simulink model "SigProcess"  (R2022b)
settings: Solver=FixedStepDiscrete  StartTime=0.0  StopTime=10.0  FixedStep=0.001  RelTol=1e-3
undefined symbols (not defined in the file): cClCddAdc_D_u16ADNum, cClCddAdc_D_u8FilterType, cClCddAdc_D_u8RawValueNum, cTmAfCtrl_Te_s32ShttrPosnColdOnHp
libraries: simulink x132
(part 5 of 7)

== system SigProcess/SigProcessSub/Stp6_createPortGotoUpdate/CLHB02001_AdFilter/AVG6 ==
  sigin : Inport
  Compare To Constant : simulink/Logic and Bit Operations/Compare To Constant  relop===  const=0  OutDataTypeStr=boolean
  Constant : Constant  Value=cClCddAdc_D_u8FilterType  OutDataTypeStr=uint8
  Constant1 : Constant  Value=cClCddAdc_D_u8RawValueNum  OutDataTypeStr=uint8
  Counter Limited : simulink/Sources/Counter Limited  uplimit=cClCddAdc_D_u8RawValueNum-1  tsamp=-1
  Data Store Memory : DataStoreMemory  DataStoreName=TempFlapFroLiFbRaw  ReadBeforeWriteMsg=warning  WriteAfterWriteMsg=warning  WriteAfterReadMsg=warning  ShowAdditionalParam=off  OutDataTypeStr=single  Dimensions=[1 20]
      settings: CopyFcn=set_param(gcbh,'ShowName','off');
  Data Store Read : DataStoreRead  DataStoreName=TempFlapFroLiFbRaw  IndexOptions=Index vector (dialog)  Indices=1  OutputSizes=1
  Data Store Write : DataStoreWrite  DataStoreName=TempFlapFroLiFbRaw  DataStoreElements=TempFlapFroLiFbRaw  EnableIndexing=on  IndexMode=Zero-based  IndexOptions=Index vector (port)  Indices=1  OutputSizes=1
  Data Type Conversion : DataTypeConversion  OutDataTypeStr=single  SaturateOnIntegerOverflow=off  RndMeth=Floor
  Gain1 : Gain  Gain=1/cClCddAdc_D_u8RawValueNum
  MATLAB Function : MATLAB Function  TreatAsAtomicUnit=on
  Multiport Switch : MultiPortSwitch  DataPortOrder=Zero-based contiguous  Inputs=5  DataPortForDefault=Additional data port  zeroidx=on  OutDataTypeStr=single  SaturateOnIntegerOverflow=off  InputSameDT=off
  Scope : Scope
  Sum of Elements1 : Sum  Inputs=+
  Switch : Switch  Criteria=u2 ~= 0  SaturateOnIntegerOverflow=off  InputSameDT=off
  Unit Delay : UnitDelay  SampleTime=-1  HasFrameUpgradeWarning=on
  sigAvg : Outport  OutDataTypeStr=single
  wires:
  Data Store Read/1 -> MATLAB Function/1(u), Sum of Elements1/1
  Sum of Elements1/1 -> Gain1/1
  Compare To Constant/1 -> Switch/2
  Switch/1 -> [sigAvgSimple], Unit Delay/1
  Gain1/1 -> Switch/1, [sigAvgQuick]
  Counter Limited/1 -> Compare To Constant/1, Data Store Write/2
  Data Type Conversion/1 -> [siginSingle], Data Store Write/1, Scope/1
  MATLAB Function/2(withoutEdge) -> [sigAvgSortWithoutEdge]
  Unit Delay/1 -> Switch/3
  MATLAB Function/1(mid) -> [sigAvgSortedMid]
  sigin/1 -> [sigin]
  [sigin] -> Data Type Conversion/1
  [sigin] -> Multiport Switch/7
  Constant/1 -> Multiport Switch/1
  [sigAvgSortedMid] -> Multiport Switch/3
  [sigAvgSortWithoutEdge] -> Multiport Switch/4
  [sigAvgSimple] -> Multiport Switch/5
  [sigAvgQuick] -> Multiport Switch/6
  [siginSingle] -> Multiport Switch/2
  Multiport Switch/1 -> [sigAvg]
  [sigAvg] -> sigAvg/1
  Constant1/1 -> MATLAB Function/2(num)

== system SigProcess/SigProcessSub/Stp6_createPortGotoUpdate/CLHB02001_AdFilter/AVG7 ==
  sigin : Inport
  Compare To Constant : simulink/Logic and Bit Operations/Compare To Constant  relop===  const=0  OutDataTypeStr=boolean
  Constant : Constant  Value=cClCddAdc_D_u8FilterType  OutDataTypeStr=uint8
  Constant1 : Constant  Value=cClCddAdc_D_u8RawValueNum  OutDataTypeStr=uint8
  Counter Limited : simulink/Sources/Counter Limited  uplimit=cClCddAdc_D_u8RawValueNum-1  tsamp=-1
  Data Store Memory : DataStoreMemory  DataStoreName=TempFlapFroRIFbRaw  ReadBeforeWriteMsg=warning  WriteAfterWriteMsg=warning  WriteAfterReadMsg=warning  ShowAdditionalParam=off  OutDataTypeStr=single  Dimensions=[1 20]
      settings: CopyFcn=set_param(gcbh,'ShowName','off');
  Data Store Read : DataStoreRead  DataStoreName=TempFlapFroRIFbRaw  IndexOptions=Index vector (dialog)  Indices=1  OutputSizes=1
  Data Store Write : DataStoreWrite  DataStoreName=TempFlapFroRIFbRaw  DataStoreElements=TempFlapFroRIFbRaw  EnableIndexing=on  IndexMode=Zero-based  IndexOptions=Index vector (port)  Indices=1  OutputSizes=1
  Data Type Conversion : DataTypeConversion  OutDataTypeStr=single  SaturateOnIntegerOverflow=off  RndMeth=Floor
  Gain1 : Gain  Gain=1/cClCddAdc_D_u8RawValueNum
  MATLAB Function : MATLAB Function  TreatAsAtomicUnit=on
  Multiport Switch : MultiPortSwitch  DataPortOrder=Zero-based contiguous  Inputs=5  DataPortForDefault=Additional data port  zeroidx=on  OutDataTypeStr=single  SaturateOnIntegerOverflow=off  InputSameDT=off
  Scope : Scope
  Sum of Elements1 : Sum  Inputs=+
  Switch : Switch  Criteria=u2 ~= 0  SaturateOnIntegerOverflow=off  InputSameDT=off
  Unit Delay : UnitDelay  SampleTime=-1  HasFrameUpgradeWarning=on
  sigAvg : Outport  OutDataTypeStr=single
  wires:
  Constant1/1 -> MATLAB Function/2(num)
  [sigAvg] -> sigAvg/1
  Multiport Switch/1 -> [sigAvg]
  [siginSingle] -> Multiport Switch/2
  [sigAvgQuick] -> Multiport Switch/6
  [sigAvgSimple] -> Multiport Switch/5
  [sigAvgSortWithoutEdge] -> Multiport Switch/4
  [sigAvgSortedMid] -> Multiport Switch/3
  Constant/1 -> Multiport Switch/1
  [sigin] -> Multiport Switch/7
  [sigin] -> Data Type Conversion/1
  sigin/1 -> [sigin]
  MATLAB Function/1(mid) -> [sigAvgSortedMid]
  Unit Delay/1 -> Switch/3
  MATLAB Function/2(withoutEdge) -> [sigAvgSortWithoutEdge]
  Data Type Conversion/1 -> Scope/1, Data Store Write/1, [siginSingle]
  Counter Limited/1 -> Data Store Write/2, Compare To Constant/1
  Gain1/1 -> [sigAvgQuick], Switch/1
  Switch/1 -> Unit Delay/1, [sigAvgSimple]
  Compare To Constant/1 -> Switch/2
  Sum of Elements1/1 -> Gain1/1
  Data Store Read/1 -> Sum of Elements1/1, MATLAB Function/1(u)

== system SigProcess/SigProcessSub/Stp6_createPortGotoUpdate/CLHB02001_AdFilter/AVG8 ==
  sigin : Inport
  Compare To Constant : simulink/Logic and Bit Operations/Compare To Constant  relop===  const=0  OutDataTypeStr=boolean
  Constant : Constant  Value=cClCddAdc_D_u8FilterType  OutDataTypeStr=uint8
  Constant1 : Constant  Value=cClCddAdc_D_u8RawValueNum  OutDataTypeStr=uint8
  Counter Limited : simulink/Sources/Counter Limited  uplimit=cClCddAdc_D_u8RawValueNum-1  tsamp=-1
  Data Store Memory : DataStoreMemory  DataStoreName=ModFlapFroRIFbRaw  ReadBeforeWriteMsg=warning  WriteAfterWriteMsg=warning  WriteAfterReadMsg=warning  ShowAdditionalParam=off  OutDataTypeStr=single  Dimensions=[1 20]
      settings: CopyFcn=set_param(gcbh,'ShowName','off');
  Data Store Read : DataStoreRead  DataStoreName=ModFlapFroRIFbRaw  IndexOptions=Index vector (dialog)  Indices=1  OutputSizes=1
  Data Store Write : DataStoreWrite  DataStoreName=ModFlapFroRIFbRaw  DataStoreElements=ModFlapFroRIFbRaw  EnableIndexing=on  IndexMode=Zero-based  IndexOptions=Index vector (port)  Indices=1  OutputSizes=1
  Data Type Conversion : DataTypeConversion  OutDataTypeStr=single  SaturateOnIntegerOverflow=off  RndMeth=Floor
  Gain1 : Gain  Gain=1/cClCddAdc_D_u8RawValueNum
  MATLAB Function : MATLAB Function  TreatAsAtomicUnit=on
  Multiport Switch : MultiPortSwitch  DataPortOrder=Zero-based contiguous  Inputs=5  DataPortForDefault=Additional data port  zeroidx=on  OutDataTypeStr=single  SaturateOnIntegerOverflow=off  InputSameDT=off
  Scope : Scope
  Sum of Elements1 : Sum  Inputs=+
  Switch : Switch  Criteria=u2 ~= 0  SaturateOnIntegerOverflow=off  InputSameDT=off
  Unit Delay : UnitDelay  SampleTime=-1  HasFrameUpgradeWarning=on
  sigAvg : Outport  OutDataTypeStr=single
  wires:
  Data Store Read/1 -> MATLAB Function/1(u), Sum of Elements1/1
  Sum of Elements1/1 -> Gain1/1
  Compare To Constant/1 -> Switch/2
  Switch/1 -> [sigAvgSimple], Unit Delay/1
  Gain1/1 -> Switch/1, [sigAvgQuick]
  Counter Limited/1 -> Compare To Constant/1, Data Store Write/2
  Data Type Conversion/1 -> [siginSingle], Data Store Write/1, Scope/1
  MATLAB Function/2(withoutEdge) -> [sigAvgSortWithoutEdge]
  Unit Delay/1 -> Switch/3
  MATLAB Function/1(mid) -> [sigAvgSortedMid]
  sigin/1 -> [sigin]
  [sigin] -> Data Type Conversion/1
  [sigin] -> Multiport Switch/7
  Constant/1 -> Multiport Switch/1
  [sigAvgSortedMid] -> Multiport Switch/3
  [sigAvgSortWithoutEdge] -> Multiport Switch/4
  [sigAvgSimple] -> Multiport Switch/5
  [sigAvgQuick] -> Multiport Switch/6
  [siginSingle] -> Multiport Switch/2
  Multiport Switch/1 -> [sigAvg]
  [sigAvg] -> sigAvg/1
  Constant1/1 -> MATLAB Function/2(num)

== system SigProcess/SigProcessSub/Stp6_createPortGotoUpdate/CLHB02001_AdFilter/AVG9 ==
  sigin : Inport
  Compare To Constant : simulink/Logic and Bit Operations/Compare To Constant  relop===  const=0  OutDataTypeStr=boolean
  Constant : Constant  Value=cClCddAdc_D_u8FilterType  OutDataTypeStr=uint8
  Constant1 : Constant  Value=cClCddAdc_D_u8RawValueNum  OutDataTypeStr=uint8
  Counter Limited : simulink/Sources/Counter Limited  uplimit=cClCddAdc_D_u8RawValueNum-1  tsamp=-1
  Data Store Memory : DataStoreMemory  DataStoreName=AqsPinRaw  ReadBeforeWriteMsg=warning  WriteAfterWriteMsg=warning  WriteAfterReadMsg=warning  ShowAdditionalParam=off  OutDataTypeStr=single  Dimensions=[1 20]
      settings: CopyFcn=set_param(gcbh,'ShowName','off');
  Data Store Read : DataStoreRead  DataStoreName=AqsPinRaw  IndexOptions=Index vector (dialog)  Indices=1  OutputSizes=1
  Data Store Write : DataStoreWrite  DataStoreName=AqsPinRaw  DataStoreElements=AqsPinRaw  EnableIndexing=on  IndexMode=Zero-based  IndexOptions=Index vector (port)  Indices=1  OutputSizes=1
  Data Type Conversion : DataTypeConversion  OutDataTypeStr=single  SaturateOnIntegerOverflow=off  RndMeth=Floor
  Gain1 : Gain  Gain=1/cClCddAdc_D_u8RawValueNum
  MATLAB Function : MATLAB Function  TreatAsAtomicUnit=on
  Multiport Switch : MultiPortSwitch  DataPortOrder=Zero-based contiguous  Inputs=5  DataPortForDefault=Additional data port  zeroidx=on  OutDataTypeStr=single  SaturateOnIntegerOverflow=off  InputSameDT=off
  Scope : Scope
  Sum of Elements1 : Sum  Inputs=+
  Switch : Switch  Criteria=u2 ~= 0  SaturateOnIntegerOverflow=off  InputSameDT=off
  Unit Delay : UnitDelay  SampleTime=-1  HasFrameUpgradeWarning=on
  sigAvg : Outport  OutDataTypeStr=single
  wires:
  Constant1/1 -> MATLAB Function/2(num)
  [sigAvg] -> sigAvg/1
  Multiport Switch/1 -> [sigAvg]
  [siginSingle] -> Multiport Switch/2
  [sigAvgQuick] -> Multiport Switch/6
  [sigAvgSimple] -> Multiport Switch/5
  [sigAvgSortWithoutEdge] -> Multiport Switch/4
  [sigAvgSortedMid] -> Multiport Switch/3
  Constant/1 -> Multiport Switch/1
  [sigin] -> Multiport Switch/7
  [sigin] -> Data Type Conversion/1
  sigin/1 -> [sigin]
  MATLAB Function/1(mid) -> [sigAvgSortedMid]
  Unit Delay/1 -> Switch/3
  MATLAB Function/2(withoutEdge) -> [sigAvgSortWithoutEdge]
  Data Type Conversion/1 -> Scope/1, Data Store Write/1, [siginSingle]
  Counter Limited/1 -> Data Store Write/2, Compare To Constant/1
  Gain1/1 -> [sigAvgQuick], Switch/1
  Switch/1 -> Unit Delay/1, [sigAvgSimple]
  Compare To Constant/1 -> Switch/2
  Sum of Elements1/1 -> Gain1/1
  Data Store Read/1 -> Sum of Elements1/1, MATLAB Function/1(u)

== system SigProcess/SigProcessSub/Stp3_createGotoUpdate/CLHB02001_AdFilter/AVG/CLHB02002_Ad2Volt ==
  ad : Inport
  Gain : Gain  Gain=5/cClCddAdc_D_u16ADNum
  volt : Outport
  wires:
  ad/1 -> Gain/1
  Gain/1 -> volt/1

== system SigProcess/SigProcessSub/Stp4_createSubModInfo/CLHB02001_AdFilter/AVG/CLHB02002_Ad2Volt ==
  ad : Inport
  Gain : Gain  Gain=5/cClCddAdc_D_u16ADNum
  volt : Outport
  wires:
  ad/1 -> Gain/1
  Gain/1 -> volt/1

== system SigProcess/SigProcessSub/Stp5_ChangeAttrAndName/1_createPortGotoUpdate/11_AdFilter/1110_AVG6 ==
  sigin : Inport
  11101_MATLAB Function : MATLAB Function  TreatAsAtomicUnit=on
  Compare To Constant : simulink/Logic and Bit Operations/Compare To Constant  relop===  const=0  OutDataTypeStr=boolean
  Constant : Constant  Value=cClCddAdc_D_u8FilterType  OutDataTypeStr=uint8
  Constant1 : Constant  Value=cClCddAdc_D_u8RawValueNum  OutDataTypeStr=uint8
  Counter Limited : simulink/Sources/Counter Limited  uplimit=cClCddAdc_D_u8RawValueNum-1  tsamp=-1
  Data Store Memory : DataStoreMemory  DataStoreName=TempFlapFroLiFbRaw  ReadBeforeWriteMsg=warning  WriteAfterWriteMsg=warning  WriteAfterReadMsg=warning  ShowAdditionalParam=off  OutDataTypeStr=single  Dimensions=[1 20]
      settings: CopyFcn=set_param(gcbh,'ShowName','off');
  Data Store Read : DataStoreRead  DataStoreName=TempFlapFroLiFbRaw  IndexOptions=Index vector (dialog)  Indices=1  OutputSizes=1
  Data Store Write : DataStoreWrite  DataStoreName=TempFlapFroLiFbRaw  DataStoreElements=TempFlapFroLiFbRaw  EnableIndexing=on  IndexMode=Zero-based  IndexOptions=Index vector (port)  Indices=1  OutputSizes=1
  Data Type Conversion : DataTypeConversion  OutDataTypeStr=single  SaturateOnIntegerOverflow=off  RndMeth=Floor
  Gain1 : Gain  Gain=1/cClCddAdc_D_u8RawValueNum
  Multiport Switch : MultiPortSwitch  DataPortOrder=Zero-based contiguous  Inputs=5  DataPortForDefault=Additional data port  zeroidx=on  OutDataTypeStr=single  SaturateOnIntegerOverflow=off  InputSameDT=off
  Scope : Scope
  Sum of Elements1 : Sum  Inputs=+
  Switch : Switch  Criteria=u2 ~= 0  SaturateOnIntegerOverflow=off  InputSameDT=off
  Unit Delay : UnitDelay  SampleTime=-1  HasFrameUpgradeWarning=on
  sigAvg : Outport  OutDataTypeStr=single
  wires:
  Data Store Read/1 -> 11101_MATLAB Function/1(u), Sum of Elements1/1
  Sum of Elements1/1 -> Gain1/1
  Compare To Constant/1 -> Switch/2
  Switch/1 -> [sigAvgSimple], Unit Delay/1
  Gain1/1 -> Switch/1, [sigAvgQuick]
  Counter Limited/1 -> Compare To Constant/1, Data Store Write/2
  Data Type Conversion/1 -> [siginSingle], Data Store Write/1, Scope/1
  11101_MATLAB Function/2(withoutEdge) -> [sigAvgSortWithoutEdge]
  Unit Delay/1 -> Switch/3
  11101_MATLAB Function/1(mid) -> [sigAvgSortedMid]
  sigin/1 -> [sigin]
  [sigin] -> Data Type Conversion/1
  [sigin] -> Multiport Switch/7
  Constant/1 -> Multiport Switch/1
  [sigAvgSortedMid] -> Multiport Switch/3
  [sigAvgSortWithoutEdge] -> Multiport Switch/4
  [sigAvgSimple] -> Multiport Switch/5
  [sigAvgQuick] -> Multiport Switch/6
  [siginSingle] -> Multiport Switch/2
  Multiport Switch/1 -> [sigAvg]
  [sigAvg] -> sigAvg/1
  Constant1/1 -> 11101_MATLAB Function/2(num)

== system SigProcess/SigProcessSub/Stp5_ChangeAttrAndName/1_createPortGotoUpdate/11_AdFilter/1111_AVG7 ==
  sigin : Inport
  11111_MATLAB Function : MATLAB Function  TreatAsAtomicUnit=on
  Compare To Constant : simulink/Logic and Bit Operations/Compare To Constant  relop===  const=0  OutDataTypeStr=boolean
  Constant : Constant  Value=cClCddAdc_D_u8FilterType  OutDataTypeStr=uint8
  Constant1 : Constant  Value=cClCddAdc_D_u8RawValueNum  OutDataTypeStr=uint8
  Counter Limited : simulink/Sources/Counter Limited  uplimit=cClCddAdc_D_u8RawValueNum-1  tsamp=-1
  Data Store Memory : DataStoreMemory  DataStoreName=TempFlapFroRIFbRaw  ReadBeforeWriteMsg=warning  WriteAfterWriteMsg=warning  WriteAfterReadMsg=warning  ShowAdditionalParam=off  OutDataTypeStr=single  Dimensions=[1 20]
      settings: CopyFcn=set_param(gcbh,'ShowName','off');
  Data Store Read : DataStoreRead  DataStoreName=TempFlapFroRIFbRaw  IndexOptions=Index vector (dialog)  Indices=1  OutputSizes=1
  Data Store Write : DataStoreWrite  DataStoreName=TempFlapFroRIFbRaw  DataStoreElements=TempFlapFroRIFbRaw  EnableIndexing=on  IndexMode=Zero-based  IndexOptions=Index vector (port)  Indices=1  OutputSizes=1
  Data Type Conversion : DataTypeConversion  OutDataTypeStr=single  SaturateOnIntegerOverflow=off  RndMeth=Floor
  Gain1 : Gain  Gain=1/cClCddAdc_D_u8RawValueNum
  Multiport Switch : MultiPortSwitch  DataPortOrder=Zero-based contiguous  Inputs=5  DataPortForDefault=Additional data port  zeroidx=on  OutDataTypeStr=single  SaturateOnIntegerOverflow=off  InputSameDT=off
  Scope : Scope
  Sum of Elements1 : Sum  Inputs=+
  Switch : Switch  Criteria=u2 ~= 0  SaturateOnIntegerOverflow=off  InputSameDT=off
  Unit Delay : UnitDelay  SampleTime=-1  HasFrameUpgradeWarning=on
  sigAvg : Outport  OutDataTypeStr=single
  wires:
  Constant1/1 -> 11111_MATLAB Function/2(num)
  [sigAvg] -> sigAvg/1
  Multiport Switch/1 -> [sigAvg]
  [siginSingle] -> Multiport Switch/2
  [sigAvgQuick] -> Multiport Switch/6
  [sigAvgSimple] -> Multiport Switch/5
  [sigAvgSortWithoutEdge] -> Multiport Switch/4
  [sigAvgSortedMid] -> Multiport Switch/3
  Constant/1 -> Multiport Switch/1
  [sigin] -> Multiport Switch/7
  [sigin] -> Data Type Conversion/1
  sigin/1 -> [sigin]
  11111_MATLAB Function/1(mid) -> [sigAvgSortedMid]
  Unit Delay/1 -> Switch/3
  11111_MATLAB Function/2(withoutEdge) -> [sigAvgSortWithoutEdge]
  Data Type Conversion/1 -> Scope/1, Data Store Write/1, [siginSingle]
  Counter Limited/1 -> Data Store Write/2, Compare To Constant/1
  Gain1/1 -> [sigAvgQuick], Switch/1
  Switch/1 -> Unit Delay/1, [sigAvgSimple]
  Compare To Constant/1 -> Switch/2
  Sum of Elements1/1 -> Gain1/1
  Data Store Read/1 -> Sum of Elements1/1, 11111_MATLAB Function/1(u)

== system SigProcess/SigProcessSub/Stp5_ChangeAttrAndName/1_createPortGotoUpdate/11_AdFilter/111_AVG8 ==
  sigin : Inport
  1111_MATLAB Function : MATLAB Function  TreatAsAtomicUnit=on
  Compare To Constant : simulink/Logic and Bit Operations/Compare To Constant  relop===  const=0  OutDataTypeStr=boolean
  Constant : Constant  Value=cClCddAdc_D_u8FilterType  OutDataTypeStr=uint8
  Constant1 : Constant  Value=cClCddAdc_D_u8RawValueNum  OutDataTypeStr=uint8
  Counter Limited : simulink/Sources/Counter Limited  uplimit=cClCddAdc_D_u8RawValueNum-1  tsamp=-1
  Data Store Memory : DataStoreMemory  DataStoreName=ModFlapFroRIFbRaw  ReadBeforeWriteMsg=warning  WriteAfterWriteMsg=warning  WriteAfterReadMsg=warning  ShowAdditionalParam=off  OutDataTypeStr=single  Dimensions=[1 20]
      settings: CopyFcn=set_param(gcbh,'ShowName','off');
  Data Store Read : DataStoreRead  DataStoreName=ModFlapFroRIFbRaw  IndexOptions=Index vector (dialog)  Indices=1  OutputSizes=1
  Data Store Write : DataStoreWrite  DataStoreName=ModFlapFroRIFbRaw  DataStoreElements=ModFlapFroRIFbRaw  EnableIndexing=on  IndexMode=Zero-based  IndexOptions=Index vector (port)  Indices=1  OutputSizes=1
  Data Type Conversion : DataTypeConversion  OutDataTypeStr=single  SaturateOnIntegerOverflow=off  RndMeth=Floor
  Gain1 : Gain  Gain=1/cClCddAdc_D_u8RawValueNum
  Multiport Switch : MultiPortSwitch  DataPortOrder=Zero-based contiguous  Inputs=5  DataPortForDefault=Additional data port  zeroidx=on  OutDataTypeStr=single  SaturateOnIntegerOverflow=off  InputSameDT=off
  Scope : Scope
  Sum of Elements1 : Sum  Inputs=+
  Switch : Switch  Criteria=u2 ~= 0  SaturateOnIntegerOverflow=off  InputSameDT=off
  Unit Delay : UnitDelay  SampleTime=-1  HasFrameUpgradeWarning=on
  sigAvg : Outport  OutDataTypeStr=single
  wires:
  Data Store Read/1 -> 1111_MATLAB Function/1(u), Sum of Elements1/1
  Sum of Elements1/1 -> Gain1/1
  Compare To Constant/1 -> Switch/2
  Switch/1 -> [sigAvgSimple], Unit Delay/1
  Gain1/1 -> Switch/1, [sigAvgQuick]
  Counter Limited/1 -> Compare To Constant/1, Data Store Write/2
  Data Type Conversion/1 -> [siginSingle], Data Store Write/1, Scope/1
  1111_MATLAB Function/2(withoutEdge) -> [sigAvgSortWithoutEdge]
  Unit Delay/1 -> Switch/3
  1111_MATLAB Function/1(mid) -> [sigAvgSortedMid]
  sigin/1 -> [sigin]
  [sigin] -> Data Type Conversion/1
  [sigin] -> Multiport Switch/7
  Constant/1 -> Multiport Switch/1
  [sigAvgSortedMid] -> Multiport Switch/3
  [sigAvgSortWithoutEdge] -> Multiport Switch/4
  [sigAvgSimple] -> Multiport Switch/5
  [sigAvgQuick] -> Multiport Switch/6
  [siginSingle] -> Multiport Switch/2
  Multiport Switch/1 -> [sigAvg]
  [sigAvg] -> sigAvg/1
  Constant1/1 -> 1111_MATLAB Function/2(num)

== system SigProcess/SigProcessSub/Stp5_ChangeAttrAndName/1_createPortGotoUpdate/11_AdFilter/112_AVG9 ==
  sigin : Inport
  1121_MATLAB Function : MATLAB Function  TreatAsAtomicUnit=on
  Compare To Constant : simulink/Logic and Bit Operations/Compare To Constant  relop===  const=0  OutDataTypeStr=boolean
  Constant : Constant  Value=cClCddAdc_D_u8FilterType  OutDataTypeStr=uint8
  Constant1 : Constant  Value=cClCddAdc_D_u8RawValueNum  OutDataTypeStr=uint8
  Counter Limited : simulink/Sources/Counter Limited  uplimit=cClCddAdc_D_u8RawValueNum-1  tsamp=-1
  Data Store Memory : DataStoreMemory  DataStoreName=AqsPinRaw  ReadBeforeWriteMsg=warning  WriteAfterWriteMsg=warning  WriteAfterReadMsg=warning  ShowAdditionalParam=off  OutDataTypeStr=single  Dimensions=[1 20]
      settings: CopyFcn=set_param(gcbh,'ShowName','off');
  Data Store Read : DataStoreRead  DataStoreName=AqsPinRaw  IndexOptions=Index vector (dialog)  Indices=1  OutputSizes=1
  Data Store Write : DataStoreWrite  DataStoreName=AqsPinRaw  DataStoreElements=AqsPinRaw  EnableIndexing=on  IndexMode=Zero-based  IndexOptions=Index vector (port)  Indices=1  OutputSizes=1
  Data Type Conversion : DataTypeConversion  OutDataTypeStr=single  SaturateOnIntegerOverflow=off  RndMeth=Floor
  Gain1 : Gain  Gain=1/cClCddAdc_D_u8RawValueNum
  Multiport Switch : MultiPortSwitch  DataPortOrder=Zero-based contiguous  Inputs=5  DataPortForDefault=Additional data port  zeroidx=on  OutDataTypeStr=single  SaturateOnIntegerOverflow=off  InputSameDT=off
  Scope : Scope
  Sum of Elements1 : Sum  Inputs=+
  Switch : Switch  Criteria=u2 ~= 0  SaturateOnIntegerOverflow=off  InputSameDT=off
  Unit Delay : UnitDelay  SampleTime=-1  HasFrameUpgradeWarning=on
  sigAvg : Outport  OutDataTypeStr=single
  wires:
  Constant1/1 -> 1121_MATLAB Function/2(num)
  [sigAvg] -> sigAvg/1
  Multiport Switch/1 -> [sigAvg]
  [siginSingle] -> Multiport Switch/2
  [sigAvgQuick] -> Multiport Switch/6
  [sigAvgSimple] -> Multiport Switch/5
  [sigAvgSortWithoutEdge] -> Multiport Switch/4
  [sigAvgSortedMid] -> Multiport Switch/3
  Constant/1 -> Multiport Switch/1
  [sigin] -> Multiport Switch/7
  [sigin] -> Data Type Conversion/1
  sigin/1 -> [sigin]
  1121_MATLAB Function/1(mid) -> [sigAvgSortedMid]
  Unit Delay/1 -> Switch/3
  1121_MATLAB Function/2(withoutEdge) -> [sigAvgSortWithoutEdge]
  Data Type Conversion/1 -> Scope/1, Data Store Write/1, [siginSingle]
  Counter Limited/1 -> Data Store Write/2, Compare To Constant/1
  Gain1/1 -> [sigAvgQuick], Switch/1
  Switch/1 -> Unit Delay/1, [sigAvgSimple]
  Compare To Constant/1 -> Switch/2
  Sum of Elements1/1 -> Gain1/1
  Data Store Read/1 -> Sum of Elements1/1, 1121_MATLAB Function/1(u)

== system SigProcess/SigProcessSub/Stp5_ChangeAttrAndName/1_createPortGotoUpdate/11_AdFilter/113_AVG ==
  note: <模型信息: AVG>
      |
      |
      | 【输入端口】
      | sigin
      |
      | 【输出端口】
      | sigAvg
      |
      | 【标定量】
      | cClCddAdc_D_u8FilterType=
      | cClCddAdc_D_u8RawValueNum=
      |
      | 创建时间: 2025-06-10 10:22:07
  sigin : Inport
  1131_Ad2Volt : Subsystem
  1132_MATLAB Function : MATLAB Function  TreatAsAtomicUnit=on
  Compare To Constant : simulink/Logic and Bit Operations/Compare To Constant  relop===  const=0  OutDataTypeStr=boolean
  Constant : Constant  Value=cClCddAdc_D_u8FilterType  OutDataTypeStr=uint8
  Constant1 : Constant  Value=cClCddAdc_D_u8RawValueNum  OutDataTypeStr=uint8
  Constant2 : Constant  Commented=on  Value=cTmAfCtrl_Te_s32ShttrPosnColdOnHp
  Counter Limited : simulink/Sources/Counter Limited  uplimit=cClCddAdc_D_u8RawValueNum-1  tsamp=-1
  Data Store Memory : DataStoreMemory  DataStoreName=BattRaw  ReadBeforeWriteMsg=warning  WriteAfterWriteMsg=warning  WriteAfterReadMsg=warning  ShowAdditionalParam=off  OutDataTypeStr=single  Dimensions=[1 20]
      settings: CopyFcn=set_param(gcbh,'ShowName','off');
  Data Store Read : DataStoreRead  DataStoreName=BattRaw  IndexOptions=Index vector (dialog)  Indices=1  OutputSizes=1
  Data Store Write : DataStoreWrite  DataStoreName=BattRaw  DataStoreElements=BattRaw  EnableIndexing=on  IndexMode=Zero-based  IndexOptions=Index vector (port)  Indices=1  OutputSizes=1
  Data Type Conversion : DataTypeConversion  OutDataTypeStr=single  SaturateOnIntegerOverflow=off  RndMeth=Floor
  Gain1 : Gain  Gain=1/cClCddAdc_D_u8RawValueNum
  Multiport Switch : MultiPortSwitch  DataPortOrder=Zero-based contiguous  Inputs=5  DataPortForDefault=Additional data port  zeroidx=on  OutDataTypeStr=single  SaturateOnIntegerOverflow=off  InputSameDT=off
  Scope : Scope
  Sum of Elements1 : Sum  Inputs=+
  Switch : Switch  Criteria=u2 ~= 0  SaturateOnIntegerOverflow=off  InputSameDT=off
  Terminator : Terminator  Commented=on
  Unit Delay : UnitDelay  SampleTime=-1  HasFrameUpgradeWarning=on
  sigAvg : Outport  OutDataTypeStr=single
  wires:
  Data Store Read/1 -> 1132_MATLAB Function/1(u), Sum of Elements1/1
  Sum of Elements1/1 -> Gain1/1
  Compare To Constant/1 -> Switch/2
  Switch/1 -> [sigAvgSimple], Unit Delay/1
  Gain1/1 -> Switch/1, [sigAvgQuick]
  Counter Limited/1 -> Compare To Constant/1, Data Store Write/2
  Data Type Conversion/1 -> [siginSingle], Data Store Write/1, Scope/1
  1132_MATLAB Function/2(withoutEdge) -> [sigAvgSortWithoutEdge]
  Unit Delay/1 -> Switch/3
  1132_MATLAB Function/1(mid) -> [sigAvgSortedMid]
  sigin/1 -> [sigin]
  [sigin] -> Data Type Conversion/1
  [sigin] -> Multiport Switch/7
  Constant/1 -> Multiport Switch/1
  [sigAvgSortedMid] -> Multiport Switch/3
  [sigAvgSortWithoutEdge] -> Multiport Switch/4
  [sigAvgSimple] -> Multiport Switch/5
  [sigAvgQuick] -> Multiport Switch/6
  [siginSingle] -> Multiport Switch/2
  Multiport Switch/1 -> 1131_Ad2Volt/1(ad)
  [sigAvg] -> sigAvg/1
  Constant1/1 -> 1132_MATLAB Function/2(num)
  1131_Ad2Volt/1(volt) -> [sigAvg]
  Constant2/1 -> Terminator/1

== system SigProcess/SigProcessSub/Stp5_ChangeAttrAndName/1_createPortGotoUpdate/11_AdFilter/114_AVG1 ==
  sigin : Inport
  1141_MATLAB Function : MATLAB Function  TreatAsAtomicUnit=on
  Compare To Constant : simulink/Logic and Bit Operations/Compare To Constant  relop===  const=0  OutDataTypeStr=boolean
  Constant : Constant  Value=cClCddAdc_D_u8FilterType  OutDataTypeStr=uint8
  Constant1 : Constant  Value=cClCddAdc_D_u8RawValueNum  OutDataTypeStr=uint8
  Counter Limited : simulink/Sources/Counter Limited  uplimit=cClCddAdc_D_u8RawValueNum-1  tsamp=-1
  Data Store Memory : DataStoreMemory  DataStoreName=EvapRaw  ReadBeforeWriteMsg=warning  WriteAfterWriteMsg=warning  WriteAfterReadMsg=warning  ShowAdditionalParam=off  OutDataTypeStr=single  Dimensions=[1 20]
      settings: CopyFcn=set_param(gcbh,'ShowName','off');
  Data Store Read : DataStoreRead  DataStoreName=EvapRaw  IndexOptions=Index vector (dialog)  Indices=1  OutputSizes=1
  Data Store Write : DataStoreWrite  DataStoreName=EvapRaw  DataStoreElements=EvapRaw  EnableIndexing=on  IndexMode=Zero-based  IndexOptions=Index vector (port)  Indices=1  OutputSizes=1
  Data Type Conversion : DataTypeConversion  OutDataTypeStr=single  SaturateOnIntegerOverflow=off  RndMeth=Floor
  Gain1 : Gain  Gain=1/cClCddAdc_D_u8RawValueNum
  Multiport Switch : MultiPortSwitch  DataPortOrder=Zero-based contiguous  Inputs=5  DataPortForDefault=Additional data port  zeroidx=on  OutDataTypeStr=single  SaturateOnIntegerOverflow=off  InputSameDT=off
  Scope : Scope
  Sum of Elements1 : Sum  Inputs=+
  Switch : Switch  Criteria=u2 ~= 0  SaturateOnIntegerOverflow=off  InputSameDT=off
  Unit Delay : UnitDelay  SampleTime=-1  HasFrameUpgradeWarning=on
  sigAvg : Outport  OutDataTypeStr=single
  wires:
  Constant1/1 -> 1141_MATLAB Function/2(num)
  [sigAvg] -> sigAvg/1
  Multiport Switch/1 -> [sigAvg]
  [siginSingle] -> Multiport Switch/2
  [sigAvgQuick] -> Multiport Switch/6
  [sigAvgSimple] -> Multiport Switch/5
  [sigAvgSortWithoutEdge] -> Multiport Switch/4
  [sigAvgSortedMid] -> Multiport Switch/3
  Constant/1 -> Multiport Switch/1
  [sigin] -> Multiport Switch/7
  [sigin] -> Data Type Conversion/1
  sigin/1 -> [sigin]
  1141_MATLAB Function/1(mid) -> [sigAvgSortedMid]
  Unit Delay/1 -> Switch/3
  1141_MATLAB Function/2(withoutEdge) -> [sigAvgSortWithoutEdge]
  Data Type Conversion/1 -> Scope/1, Data Store Write/1, [siginSingle]
  Counter Limited/1 -> Data Store Write/2, Compare To Constant/1
  Gain1/1 -> [sigAvgQuick], Switch/1
  Switch/1 -> Unit Delay/1, [sigAvgSimple]
  Compare To Constant/1 -> Switch/2
  Sum of Elements1/1 -> Gain1/1
  Data Store Read/1 -> Sum of Elements1/1, 1141_MATLAB Function/1(u)

== system SigProcess/SigProcessSub/Stp5_ChangeAttrAndName/1_createPortGotoUpdate/11_AdFilter/115_AVG10 ==
  sigin : Inport
  1151_MATLAB Function : MATLAB Function  TreatAsAtomicUnit=on
  Compare To Constant : simulink/Logic and Bit Operations/Compare To Constant  relop===  const=0  OutDataTypeStr=boolean
  Constant : Constant  Value=cClCddAdc_D_u8FilterType  OutDataTypeStr=uint8
  Constant1 : Constant  Value=cClCddAdc_D_u8RawValueNum  OutDataTypeStr=uint8
  Counter Limited : simulink/Sources/Counter Limited  uplimit=cClCddAdc_D_u8RawValueNum-1  tsamp=-1
  Data Store Memory : DataStoreMemory  DataStoreName=BlowPositivePinRaw  ReadBeforeWriteMsg=warning  WriteAfterWriteMsg=warning  WriteAfterReadMsg=warning  ShowAdditionalParam=off  OutDataTypeStr=single  Dimensions=[1 20]
      settings: CopyFcn=set_param(gcbh,'ShowName','off');
  Data Store Read : DataStoreRead  DataStoreName=BlowPositivePinRaw  IndexOptions=Index vector (dialog)  Indices=1  OutputSizes=1
  Data Store Write : DataStoreWrite  DataStoreName=BlowPositivePinRaw  DataStoreElements=BlowPositivePinRaw  EnableIndexing=on  IndexMode=Zero-based  IndexOptions=Index vector (port)  Indices=1  OutputSizes=1
  Data Type Conversion : DataTypeConversion  OutDataTypeStr=single  SaturateOnIntegerOverflow=off  RndMeth=Floor
  Gain1 : Gain  Gain=1/cClCddAdc_D_u8RawValueNum
  Multiport Switch : MultiPortSwitch  DataPortOrder=Zero-based contiguous  Inputs=5  DataPortForDefault=Additional data port  zeroidx=on  OutDataTypeStr=single  SaturateOnIntegerOverflow=off  InputSameDT=off
  Scope : Scope
  Sum of Elements1 : Sum  Inputs=+
  Switch : Switch  Criteria=u2 ~= 0  SaturateOnIntegerOverflow=off  InputSameDT=off
  Unit Delay : UnitDelay  SampleTime=-1  HasFrameUpgradeWarning=on
  sigAvg : Outport  OutDataTypeStr=single
  wires:
  Data Store Read/1 -> 1151_MATLAB Function/1(u), Sum of Elements1/1
  Sum of Elements1/1 -> Gain1/1
  Compare To Constant/1 -> Switch/2
  Switch/1 -> [sigAvgSimple], Unit Delay/1
  Gain1/1 -> Switch/1, [sigAvgQuick]
  Counter Limited/1 -> Compare To Constant/1, Data Store Write/2
  Data Type Conversion/1 -> [siginSingle], Data Store Write/1, Scope/1
  1151_MATLAB Function/2(withoutEdge) -> [sigAvgSortWithoutEdge]
  Unit Delay/1 -> Switch/3
  1151_MATLAB Function/1(mid) -> [sigAvgSortedMid]
  sigin/1 -> [sigin]
  [sigin] -> Data Type Conversion/1
  [sigin] -> Multiport Switch/7
  Constant/1 -> Multiport Switch/1
  [sigAvgSortedMid] -> Multiport Switch/3
  [sigAvgSortWithoutEdge] -> Multiport Switch/4
  [sigAvgSimple] -> Multiport Switch/5
  [sigAvgQuick] -> Multiport Switch/6
  [siginSingle] -> Multiport Switch/2
  Multiport Switch/1 -> [sigAvg]
  [sigAvg] -> sigAvg/1
  Constant1/1 -> 1151_MATLAB Function/2(num)

== system SigProcess/SigProcessSub/Stp5_ChangeAttrAndName/1_createPortGotoUpdate/11_AdFilter/116_AVG2 ==
  sigin : Inport
  1161_MATLAB Function : MATLAB Function  TreatAsAtomicUnit=on
  Compare To Constant : simulink/Logic and Bit Operations/Compare To Constant  relop===  const=0  OutDataTypeStr=boolean
  Constant : Constant  Value=cClCddAdc_D_u8FilterType  OutDataTypeStr=uint8
  Constant1 : Constant  Value=cClCddAdc_D_u8RawValueNum  OutDataTypeStr=uint8
  Counter Limited : simulink/Sources/Counter Limited  uplimit=cClCddAdc_D_u8RawValueNum-1  tsamp=-1
  Data Store Memory : DataStoreMemory  DataStoreName=BlowNegativePinRaw  ReadBeforeWriteMsg=warning  WriteAfterWriteMsg=warning  WriteAfterReadMsg=warning  ShowAdditionalParam=off  OutDataTypeStr=single  Dimensions=[1 20]
      settings: CopyFcn=set_param(gcbh,'ShowName','off');
  Data Store Read : DataStoreRead  DataStoreName=BlowNegativePinRaw  IndexOptions=Index vector (dialog)  Indices=1  OutputSizes=1
  Data Store Write : DataStoreWrite  DataStoreName=BlowNegativePinRaw  DataStoreElements=BlowNegativePinRaw  EnableIndexing=on  IndexMode=Zero-based  IndexOptions=Index vector (port)  Indices=1  OutputSizes=1
  Data Type Conversion : DataTypeConversion  OutDataTypeStr=single  SaturateOnIntegerOverflow=off  RndMeth=Floor
  Gain1 : Gain  Gain=1/cClCddAdc_D_u8RawValueNum
  Multiport Switch : MultiPortSwitch  DataPortOrder=Zero-based contiguous  Inputs=5  DataPortForDefault=Additional data port  zeroidx=on  OutDataTypeStr=single  SaturateOnIntegerOverflow=off  InputSameDT=off
  Scope : Scope
  Sum of Elements1 : Sum  Inputs=+
  Switch : Switch  Criteria=u2 ~= 0  SaturateOnIntegerOverflow=off  InputSameDT=off
  Unit Delay : UnitDelay  SampleTime=-1  HasFrameUpgradeWarning=on
  sigAvg : Outport  OutDataTypeStr=single
  wires:
  Data Store Read/1 -> 1161_MATLAB Function/1(u), Sum of Elements1/1
  Sum of Elements1/1 -> Gain1/1
  Compare To Constant/1 -> Switch/2
  Switch/1 -> [sigAvgSimple], Unit Delay/1
  Gain1/1 -> Switch/1, [sigAvgQuick]
  Counter Limited/1 -> Compare To Constant/1, Data Store Write/2
  Data Type Conversion/1 -> [siginSingle], Data Store Write/1, Scope/1
  1161_MATLAB Function/2(withoutEdge) -> [sigAvgSortWithoutEdge]
  Unit Delay/1 -> Switch/3
  1161_MATLAB Function/1(mid) -> [sigAvgSortedMid]
  sigin/1 -> [sigin]
  [sigin] -> Data Type Conversion/1
  [sigin] -> Multiport Switch/7
  Constant/1 -> Multiport Switch/1
  [sigAvgSortedMid] -> Multiport Switch/3
  [sigAvgSortWithoutEdge] -> Multiport Switch/4
  [sigAvgSimple] -> Multiport Switch/5
  [sigAvgQuick] -> Multiport Switch/6
  [siginSingle] -> Multiport Switch/2
  Multiport Switch/1 -> [sigAvg]
  [sigAvg] -> sigAvg/1
  Constant1/1 -> 1161_MATLAB Function/2(num)

== system SigProcess/SigProcessSub/Stp5_ChangeAttrAndName/1_createPortGotoUpdate/11_AdFilter/117_AVG3 ==
  sigin : Inport
  1171_MATLAB Function : MATLAB Function  TreatAsAtomicUnit=on
  Compare To Constant : simulink/Logic and Bit Operations/Compare To Constant  relop===  const=0  OutDataTypeStr=boolean
  Constant : Constant  Value=cClCddAdc_D_u8FilterType  OutDataTypeStr=uint8
  Constant1 : Constant  Value=cClCddAdc_D_u8RawValueNum  OutDataTypeStr=uint8
  Counter Limited : simulink/Sources/Counter Limited  uplimit=cClCddAdc_D_u8RawValueNum-1  tsamp=-1
  Data Store Memory : DataStoreMemory  DataStoreName=HexRaw  ReadBeforeWriteMsg=warning  WriteAfterWriteMsg=warning  WriteAfterReadMsg=warning  ShowAdditionalParam=off  OutDataTypeStr=single  Dimensions=[1 20]
      settings: CopyFcn=set_param(gcbh,'ShowName','off');
  Data Store Read : DataStoreRead  DataStoreName=HexRaw  IndexOptions=Index vector (dialog)  Indices=1  OutputSizes=1
  Data Store Write : DataStoreWrite  DataStoreName=HexRaw  DataStoreElements=HexRaw  EnableIndexing=on  IndexMode=Zero-based  IndexOptions=Index vector (port)  Indices=1  OutputSizes=1
  Data Type Conversion : DataTypeConversion  OutDataTypeStr=single  SaturateOnIntegerOverflow=off  RndMeth=Floor
  Gain1 : Gain  Gain=1/cClCddAdc_D_u8RawValueNum
  Multiport Switch : MultiPortSwitch  DataPortOrder=Zero-based contiguous  Inputs=5  DataPortForDefault=Additional data port  zeroidx=on  OutDataTypeStr=single  SaturateOnIntegerOverflow=off  InputSameDT=off
  Scope : Scope
  Sum of Elements1 : Sum  Inputs=+
  Switch : Switch  Criteria=u2 ~= 0  SaturateOnIntegerOverflow=off  InputSameDT=off
  Unit Delay : UnitDelay  SampleTime=-1  HasFrameUpgradeWarning=on
  sigAvg : Outport  OutDataTypeStr=single
  wires:
  Constant1/1 -> 1171_MATLAB Function/2(num)
  [sigAvg] -> sigAvg/1
  Multiport Switch/1 -> [sigAvg]
  [siginSingle] -> Multiport Switch/2
  [sigAvgQuick] -> Multiport Switch/6
  [sigAvgSimple] -> Multiport Switch/5
  [sigAvgSortWithoutEdge] -> Multiport Switch/4
  [sigAvgSortedMid] -> Multiport Switch/3
  Constant/1 -> Multiport Switch/1
  [sigin] -> Multiport Switch/7
  [sigin] -> Data Type Conversion/1
  sigin/1 -> [sigin]
  1171_MATLAB Function/1(mid) -> [sigAvgSortedMid]
  Unit Delay/1 -> Switch/3
  1171_MATLAB Function/2(withoutEdge) -> [sigAvgSortWithoutEdge]
  Data Type Conversion/1 -> Scope/1, Data Store Write/1, [siginSingle]
  Counter Limited/1 -> Data Store Write/2, Compare To Constant/1
  Gain1/1 -> [sigAvgQuick], Switch/1
  Switch/1 -> Unit Delay/1, [sigAvgSimple]
  Compare To Constant/1 -> Switch/2
  Sum of Elements1/1 -> Gain1/1
  Data Store Read/1 -> Sum of Elements1/1, 1171_MATLAB Function/1(u)

== system SigProcess/SigProcessSub/Stp5_ChangeAttrAndName/1_createPortGotoUpdate/11_AdFilter/118_AVG4 ==
  sigin : Inport
  1181_MATLAB Function : MATLAB Function  TreatAsAtomicUnit=on
  Compare To Constant : simulink/Logic and Bit Operations/Compare To Constant  relop===  const=0  OutDataTypeStr=boolean
  Constant : Constant  Value=cClCddAdc_D_u8FilterType  OutDataTypeStr=uint8
  Constant1 : Constant  Value=cClCddAdc_D_u8RawValueNum  OutDataTypeStr=uint8
  Counter Limited : simulink/Sources/Counter Limited  uplimit=cClCddAdc_D_u8RawValueNum-1  tsamp=-1
  Data Store Memory : DataStoreMemory  DataStoreName=FroInCarRaw  ReadBeforeWriteMsg=warning  WriteAfterWriteMsg=warning  WriteAfterReadMsg=warning  ShowAdditionalParam=off  OutDataTypeStr=single  Dimensions=[1 20]
      settings: CopyFcn=set_param(gcbh,'ShowName','off');
  Data Store Read : DataStoreRead  DataStoreName=FroInCarRaw  IndexOptions=Index vector (dialog)  Indices=1  OutputSizes=1
  Data Store Write : DataStoreWrite  DataStoreName=FroInCarRaw  DataStoreElements=FroInCarRaw  EnableIndexing=on  IndexMode=Zero-based  IndexOptions=Index vector (port)  Indices=1  OutputSizes=1
  Data Type Conversion : DataTypeConversion  OutDataTypeStr=single  SaturateOnIntegerOverflow=off  RndMeth=Floor
  Gain1 : Gain  Gain=1/cClCddAdc_D_u8RawValueNum
  Multiport Switch : MultiPortSwitch  DataPortOrder=Zero-based contiguous  Inputs=5  DataPortForDefault=Additional data port  zeroidx=on  OutDataTypeStr=single  SaturateOnIntegerOverflow=off  InputSameDT=off
  Scope : Scope
  Sum of Elements1 : Sum  Inputs=+
  Switch : Switch  Criteria=u2 ~= 0  SaturateOnIntegerOverflow=off  InputSameDT=off
  Unit Delay : UnitDelay  SampleTime=-1  HasFrameUpgradeWarning=on
  sigAvg : Outport  OutDataTypeStr=single
  wires:
  Data Store Read/1 -> 1181_MATLAB Function/1(u), Sum of Elements1/1
  Sum of Elements1/1 -> Gain1/1
  Compare To Constant/1 -> Switch/2
  Switch/1 -> [sigAvgSimple], Unit Delay/1
  Gain1/1 -> Switch/1, [sigAvgQuick]
  Counter Limited/1 -> Compare To Constant/1, Data Store Write/2
  Data Type Conversion/1 -> [siginSingle], Data Store Write/1, Scope/1
  1181_MATLAB Function/2(withoutEdge) -> [sigAvgSortWithoutEdge]
  Unit Delay/1 -> Switch/3
  1181_MATLAB Function/1(mid) -> [sigAvgSortedMid]
  sigin/1 -> [sigin]
  [sigin] -> Data Type Conversion/1
  [sigin] -> Multiport Switch/7
  Constant/1 -> Multiport Switch/1
  [sigAvgSortedMid] -> Multiport Switch/3
  [sigAvgSortWithoutEdge] -> Multiport Switch/4
  [sigAvgSimple] -> Multiport Switch/5
  [sigAvgQuick] -> Multiport Switch/6
  [siginSingle] -> Multiport Switch/2
  Multiport Switch/1 -> [sigAvg]
  [sigAvg] -> sigAvg/1
  Constant1/1 -> 1181_MATLAB Function/2(num)

== system SigProcess/SigProcessSub/Stp5_ChangeAttrAndName/1_createPortGotoUpdate/11_AdFilter/119_AVG5 ==
  sigin : Inport
  1191_MATLAB Function : MATLAB Function  TreatAsAtomicUnit=on
  Compare To Constant : simulink/Logic and Bit Operations/Compare To Constant  relop===  const=0  OutDataTypeStr=boolean
  Constant : Constant  Value=cClCddAdc_D_u8FilterType  OutDataTypeStr=uint8
  Constant1 : Constant  Value=cClCddAdc_D_u8RawValueNum  OutDataTypeStr=uint8
  Counter Limited : simulink/Sources/Counter Limited  uplimit=cClCddAdc_D_u8RawValueNum-1  tsamp=-1
  Data Store Memory : DataStoreMemory  DataStoreName=RecFlapFbRaw  ReadBeforeWriteMsg=warning  WriteAfterWriteMsg=warning  WriteAfterReadMsg=warning  ShowAdditionalParam=off  OutDataTypeStr=single  Dimensions=[1 20]
      settings: CopyFcn=set_param(gcbh,'ShowName','off');
  Data Store Read : DataStoreRead  DataStoreName=RecFlapFbRaw  IndexOptions=Index vector (dialog)  Indices=1  OutputSizes=1
  Data Store Write : DataStoreWrite  DataStoreName=RecFlapFbRaw  DataStoreElements=RecFlapFbRaw  EnableIndexing=on  IndexMode=Zero-based  IndexOptions=Index vector (port)  Indices=1  OutputSizes=1
  Data Type Conversion : DataTypeConversion  OutDataTypeStr=single  SaturateOnIntegerOverflow=off  RndMeth=Floor
  Gain1 : Gain  Gain=1/cClCddAdc_D_u8RawValueNum
  Multiport Switch : MultiPortSwitch  DataPortOrder=Zero-based contiguous  Inputs=5  DataPortForDefault=Additional data port  zeroidx=on  OutDataTypeStr=single  SaturateOnIntegerOverflow=off  InputSameDT=off
  Scope : Scope
  Sum of Elements1 : Sum  Inputs=+
  Switch : Switch  Criteria=u2 ~= 0  SaturateOnIntegerOverflow=off  InputSameDT=off
  Unit Delay : UnitDelay  SampleTime=-1  HasFrameUpgradeWarning=on
  sigAvg : Outport  OutDataTypeStr=single
  wires:
  Constant1/1 -> 1191_MATLAB Function/2(num)
  [sigAvg] -> sigAvg/1
  Multiport Switch/1 -> [sigAvg]
  [siginSingle] -> Multiport Switch/2
  [sigAvgQuick] -> Multiport Switch/6
  [sigAvgSimple] -> Multiport Switch/5
  [sigAvgSortWithoutEdge] -> Multiport Switch/4
  [sigAvgSortedMid] -> Multiport Switch/3
  Constant/1 -> Multiport Switch/1
  [sigin] -> Multiport Switch/7
  [sigin] -> Data Type Conversion/1
  sigin/1 -> [sigin]
  1191_MATLAB Function/1(mid) -> [sigAvgSortedMid]
  Unit Delay/1 -> Switch/3
  1191_MATLAB Function/2(withoutEdge) -> [sigAvgSortWithoutEdge]
  Data Type Conversion/1 -> Scope/1, Data Store Write/1, [siginSingle]
  Counter Limited/1 -> Data Store Write/2, Compare To Constant/1
  Gain1/1 -> [sigAvgQuick], Switch/1
  Switch/1 -> Unit Delay/1, [sigAvgSimple]
  Compare To Constant/1 -> Switch/2
  Sum of Elements1/1 -> Gain1/1
  Data Store Read/1 -> Sum of Elements1/1, 1191_MATLAB Function/1(u)

== system SigProcess/SigProcessSub/Stp5_ChangeAttrAndName/2_createPortGotoUpdate1/21_AdFilter/2110_AVG6 ==
  sigin : Inport
  21101_MATLAB Function : MATLAB Function  TreatAsAtomicUnit=on
  Compare To Constant : simulink/Logic and Bit Operations/Compare To Constant  relop===  const=0  OutDataTypeStr=boolean
  Constant : Constant  Value=cClCddAdc_D_u8FilterType  OutDataTypeStr=uint8
  Constant1 : Constant  Value=cClCddAdc_D_u8RawValueNum  OutDataTypeStr=uint8
  Counter Limited : simulink/Sources/Counter Limited  uplimit=cClCddAdc_D_u8RawValueNum-1  tsamp=-1
  Data Store Memory : DataStoreMemory  DataStoreName=TempFlapFroLiFbRaw  ReadBeforeWriteMsg=warning  WriteAfterWriteMsg=warning  WriteAfterReadMsg=warning  ShowAdditionalParam=off  OutDataTypeStr=single  Dimensions=[1 20]
      settings: CopyFcn=set_param(gcbh,'ShowName','off');
  Data Store Read : DataStoreRead  DataStoreName=TempFlapFroLiFbRaw  IndexOptions=Index vector (dialog)  Indices=1  OutputSizes=1
  Data Store Write : DataStoreWrite  DataStoreName=TempFlapFroLiFbRaw  DataStoreElements=TempFlapFroLiFbRaw  EnableIndexing=on  IndexMode=Zero-based  IndexOptions=Index vector (port)  Indices=1  OutputSizes=1
  Data Type Conversion : DataTypeConversion  OutDataTypeStr=single  SaturateOnIntegerOverflow=off  RndMeth=Floor
  Gain1 : Gain  Gain=1/cClCddAdc_D_u8RawValueNum
  Multiport Switch : MultiPortSwitch  DataPortOrder=Zero-based contiguous  Inputs=5  DataPortForDefault=Additional data port  zeroidx=on  OutDataTypeStr=single  SaturateOnIntegerOverflow=off  InputSameDT=off
  Scope : Scope
  Sum of Elements1 : Sum  Inputs=+
  Switch : Switch  Criteria=u2 ~= 0  SaturateOnIntegerOverflow=off  InputSameDT=off
  Unit Delay : UnitDelay  SampleTime=-1  HasFrameUpgradeWarning=on
  sigAvg : Outport  OutDataTypeStr=single
  wires:
  Constant1/1 -> 21101_MATLAB Function/2(num)
  [sigAvg] -> sigAvg/1
  Multiport Switch/1 -> [sigAvg]
  [siginSingle] -> Multiport Switch/2
  [sigAvgQuick] -> Multiport Switch/6
  [sigAvgSimple] -> Multiport Switch/5
  [sigAvgSortWithoutEdge] -> Multiport Switch/4
  [sigAvgSortedMid] -> Multiport Switch/3
  Constant/1 -> Multiport Switch/1
  [sigin] -> Multiport Switch/7
  [sigin] -> Data Type Conversion/1
  sigin/1 -> [sigin]
  21101_MATLAB Function/1(mid) -> [sigAvgSortedMid]
  Unit Delay/1 -> Switch/3
  21101_MATLAB Function/2(withoutEdge) -> [sigAvgSortWithoutEdge]
  Data Type Conversion/1 -> Scope/1, Data Store Write/1, [siginSingle]
  Counter Limited/1 -> Data Store Write/2, Compare To Constant/1
  Gain1/1 -> [sigAvgQuick], Switch/1
  Switch/1 -> Unit Delay/1, [sigAvgSimple]
  Compare To Constant/1 -> Switch/2
  Sum of Elements1/1 -> Gain1/1
  Data Store Read/1 -> Sum of Elements1/1, 21101_MATLAB Function/1(u)

== system SigProcess/SigProcessSub/Stp5_ChangeAttrAndName/2_createPortGotoUpdate1/21_AdFilter/2111_AVG7 ==
  sigin : Inport
  21111_MATLAB Function : MATLAB Function  TreatAsAtomicUnit=on
  Compare To Constant : simulink/Logic and Bit Operations/Compare To Constant  relop===  const=0  OutDataTypeStr=boolean
  Constant : Constant  Value=cClCddAdc_D_u8FilterType  OutDataTypeStr=uint8
  Constant1 : Constant  Value=cClCddAdc_D_u8RawValueNum  OutDataTypeStr=uint8
  Counter Limited : simulink/Sources/Counter Limited  uplimit=cClCddAdc_D_u8RawValueNum-1  tsamp=-1
  Data Store Memory : DataStoreMemory  DataStoreName=TempFlapFroRIFbRaw  ReadBeforeWriteMsg=warning  WriteAfterWriteMsg=warning  WriteAfterReadMsg=warning  ShowAdditionalParam=off  OutDataTypeStr=single  Dimensions=[1 20]
      settings: CopyFcn=set_param(gcbh,'ShowName','off');
  Data Store Read : DataStoreRead  DataStoreName=TempFlapFroRIFbRaw  IndexOptions=Index vector (dialog)  Indices=1  OutputSizes=1
  Data Store Write : DataStoreWrite  DataStoreName=TempFlapFroRIFbRaw  DataStoreElements=TempFlapFroRIFbRaw  EnableIndexing=on  IndexMode=Zero-based  IndexOptions=Index vector (port)  Indices=1  OutputSizes=1
  Data Type Conversion : DataTypeConversion  OutDataTypeStr=single  SaturateOnIntegerOverflow=off  RndMeth=Floor
  Gain1 : Gain  Gain=1/cClCddAdc_D_u8RawValueNum
  Multiport Switch : MultiPortSwitch  DataPortOrder=Zero-based contiguous  Inputs=5  DataPortForDefault=Additional data port  zeroidx=on  OutDataTypeStr=single  SaturateOnIntegerOverflow=off  InputSameDT=off
  Scope : Scope
  Sum of Elements1 : Sum  Inputs=+
  Switch : Switch  Criteria=u2 ~= 0  SaturateOnIntegerOverflow=off  InputSameDT=off
  Unit Delay : UnitDelay  SampleTime=-1  HasFrameUpgradeWarning=on
  sigAvg : Outport  OutDataTypeStr=single
  wires:
  Data Store Read/1 -> 21111_MATLAB Function/1(u), Sum of Elements1/1
  Sum of Elements1/1 -> Gain1/1
  Compare To Constant/1 -> Switch/2
  Switch/1 -> [sigAvgSimple], Unit Delay/1
  Gain1/1 -> Switch/1, [sigAvgQuick]
  Counter Limited/1 -> Compare To Constant/1, Data Store Write/2
  Data Type Conversion/1 -> [siginSingle], Data Store Write/1, Scope/1
  21111_MATLAB Function/2(withoutEdge) -> [sigAvgSortWithoutEdge]
  Unit Delay/1 -> Switch/3
  21111_MATLAB Function/1(mid) -> [sigAvgSortedMid]
  sigin/1 -> [sigin]
  [sigin] -> Data Type Conversion/1
  [sigin] -> Multiport Switch/7
  Constant/1 -> Multiport Switch/1
  [sigAvgSortedMid] -> Multiport Switch/3
  [sigAvgSortWithoutEdge] -> Multiport Switch/4
  [sigAvgSimple] -> Multiport Switch/5
  [sigAvgQuick] -> Multiport Switch/6
  [siginSingle] -> Multiport Switch/2
  Multiport Switch/1 -> [sigAvg]
  [sigAvg] -> sigAvg/1
  Constant1/1 -> 21111_MATLAB Function/2(num)

== system SigProcess/SigProcessSub/Stp5_ChangeAttrAndName/2_createPortGotoUpdate1/21_AdFilter/211_AVG8 ==
  sigin : Inport
  2111_MATLAB Function : MATLAB Function  TreatAsAtomicUnit=on
  Compare To Constant : simulink/Logic and Bit Operations/Compare To Constant  relop===  const=0  OutDataTypeStr=boolean
  Constant : Constant  Value=cClCddAdc_D_u8FilterType  OutDataTypeStr=uint8
  Constant1 : Constant  Value=cClCddAdc_D_u8RawValueNum  OutDataTypeStr=uint8
  Counter Limited : simulink/Sources/Counter Limited  uplimit=cClCddAdc_D_u8RawValueNum-1  tsamp=-1
  Data Store Memory : DataStoreMemory  DataStoreName=ModFlapFroRIFbRaw  ReadBeforeWriteMsg=warning  WriteAfterWriteMsg=warning  WriteAfterReadMsg=warning  ShowAdditionalParam=off  OutDataTypeStr=single  Dimensions=[1 20]
      settings: CopyFcn=set_param(gcbh,'ShowName','off');
  Data Store Read : DataStoreRead  DataStoreName=ModFlapFroRIFbRaw  IndexOptions=Index vector (dialog)  Indices=1  OutputSizes=1
  Data Store Write : DataStoreWrite  DataStoreName=ModFlapFroRIFbRaw  DataStoreElements=ModFlapFroRIFbRaw  EnableIndexing=on  IndexMode=Zero-based  IndexOptions=Index vector (port)  Indices=1  OutputSizes=1
  Data Type Conversion : DataTypeConversion  OutDataTypeStr=single  SaturateOnIntegerOverflow=off  RndMeth=Floor
  Gain1 : Gain  Gain=1/cClCddAdc_D_u8RawValueNum
  Multiport Switch : MultiPortSwitch  DataPortOrder=Zero-based contiguous  Inputs=5  DataPortForDefault=Additional data port  zeroidx=on  OutDataTypeStr=single  SaturateOnIntegerOverflow=off  InputSameDT=off
  Scope : Scope
  Sum of Elements1 : Sum  Inputs=+
  Switch : Switch  Criteria=u2 ~= 0  SaturateOnIntegerOverflow=off  InputSameDT=off
  Unit Delay : UnitDelay  SampleTime=-1  HasFrameUpgradeWarning=on
  sigAvg : Outport  OutDataTypeStr=single
  wires:
  Constant1/1 -> 2111_MATLAB Function/2(num)
  [sigAvg] -> sigAvg/1
  Multiport Switch/1 -> [sigAvg]
  [siginSingle] -> Multiport Switch/2
  [sigAvgQuick] -> Multiport Switch/6
  [sigAvgSimple] -> Multiport Switch/5
  [sigAvgSortWithoutEdge] -> Multiport Switch/4
  [sigAvgSortedMid] -> Multiport Switch/3
  Constant/1 -> Multiport Switch/1
  [sigin] -> Multiport Switch/7
  [sigin] -> Data Type Conversion/1
  sigin/1 -> [sigin]
  2111_MATLAB Function/1(mid) -> [sigAvgSortedMid]
  Unit Delay/1 -> Switch/3
  2111_MATLAB Function/2(withoutEdge) -> [sigAvgSortWithoutEdge]
  Data Type Conversion/1 -> Scope/1, Data Store Write/1, [siginSingle]
  Counter Limited/1 -> Data Store Write/2, Compare To Constant/1
  Gain1/1 -> [sigAvgQuick], Switch/1
  Switch/1 -> Unit Delay/1, [sigAvgSimple]
  Compare To Constant/1 -> Switch/2
  Sum of Elements1/1 -> Gain1/1
  Data Store Read/1 -> Sum of Elements1/1, 2111_MATLAB Function/1(u)
